simulink model "bot_demo_org"  (Simulink 10.0)
settings: Solver=ode45  StartTime=0.0  StopTime=inf  FixedStep=0.1  RelTol=1e-3
undefined symbols (not defined in the file): C_l_be, C_l_p, C_l_r, C_l_xi, C_l_ze, C_Q_be, C_Q_p, C_Q_r, C_Q_xi, C_Q_ze
settings Model: Creator=jjbuchholz  LastModifiedBy=annonymous  ExtModeTrigMode=oneshot  ExtModeArmWhenConnect=off
settings DataIOCC: ExternalInput=[0 43068.267045196386 0 -0.018368082169447898 0 199.99999999999997 0 0.05890055295549914 0 0 0]  FinalStateName=xfinal  InitialState=[0;0.05890055295549914;0;0;0;0;199.65317277347208;0;11.773300365067556;0;0;0;0;0;0;43068.267045196386;43068.267045196386;43068.267045196386;43068.267045196386]  LoadExternalInput=on  LoadInitialState=on  SignalLoggingSaveFormat=ModelDataLogs  SignalLoggingName=sigsOut
settings OptimizationCC: BlockReduction=off  BooleanDataType=off  ExpressionDepthLimit=2147483647
settings DebuggingCC: SaveWithParameterizedLinksMsg=none  SignalResolutionControl=TryResolveAllWithWarning  MultiTaskDSMMsg=warning  MultiTaskCondExecSysMsg=none  FcnCallInpInsideContextMsg=warning  StateNameClashWarn=warning  InitInArrayFormatMsg=none
settings HardwareCC: TargetUnknown=on
settings GRTTargetCC: GeneratePreprocessorConditionals=Disable all
settings ConfigComp: CovExternalEMLEnable=off

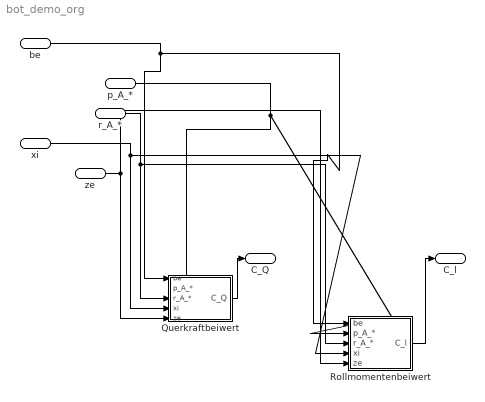
== system bot_demo_org ==
  be : Inport
  p_A_* : Inport  Port=2
  r_A_* : Inport  Port=3
  xi : Inport  Port=4
  ze : Inport  Port=5
  Querkraftbeiwert : Subsystem
  Rollmomentenbeiwert : Subsystem
  C_Q : Outport  InitialOutput=0
  C_l : Outport  Port=2  InitialOutput=0
  wires:
  Querkraftbeiwert/1(C_Q) -> C_Q/1
  Rollmomentenbeiwert/1(C_l) -> C_l/1
  ze/1 -> Querkraftbeiwert/5(ze), Rollmomentenbeiwert/5(ze)
  xi/1 -> Rollmomentenbeiwert/4(xi), Querkraftbeiwert/4(xi)
  r_A_*/1 -> Querkraftbeiwert/3(r_A_*), Rollmomentenbeiwert/3(r_A_*)
  p_A_*/1 -> Rollmomentenbeiwert/2(p_A_*), Querkraftbeiwert/2(p_A_*)
  be/1 -> Querkraftbeiwert/1(be), Rollmomentenbeiwert/1(be)

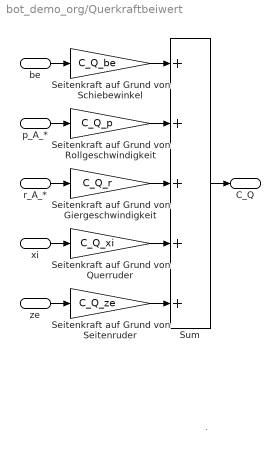
== system bot_demo_org/Querkraftbeiwert ==
  note: .
  be : Inport
  p_A_* : Inport  Port=2
  r_A_* : Inport  Port=3
  xi : Inport  Port=4
  ze : Inport  Port=5
  Seitenkraft auf Grund von Giergeschwindigkeit : Gain  Gain=C_Q_r  SaturateOnIntegerOverflow=on  OutDataTypeStr=Inherit: Same as input  ParamDataTypeStr=Inherit: Same as input
  Seitenkraft auf Grund von Querruder : Gain  Gain=C_Q_xi  SaturateOnIntegerOverflow=on  OutDataTypeStr=Inherit: Same as input  ParamDataTypeStr=Inherit: Same as input
  Seitenkraft auf Grund von Rollgeschwindigkeit : Gain  Gain=C_Q_p  SaturateOnIntegerOverflow=on  OutDataTypeStr=Inherit: Same as input  ParamDataTypeStr=Inherit: Same as input
  Seitenkraft auf Grund von Schiebewinkel : Gain  Gain=C_Q_be  SaturateOnIntegerOverflow=on  OutDataTypeStr=Inherit: Same as input  ParamDataTypeStr=Inherit: Same as input
  Seitenkraft auf Grund von Seitenruder : Gain  Gain=C_Q_ze  SaturateOnIntegerOverflow=on  OutDataTypeStr=Inherit: Same as input  ParamDataTypeStr=Inherit: Same as input
  Sum : Sum  Inputs=5  SaturateOnIntegerOverflow=on  InputSameDT=on  OutDataTypeStr=Inherit: Same as first input
  C_Q : Outport  InitialOutput=0
  wires:
  xi/1 -> Seitenkraft auf Grund von Querruder/1
  r_A_*/1 -> Seitenkraft auf Grund von Giergeschwindigkeit/1
  Sum/1 -> C_Q/1
  p_A_*/1 -> Seitenkraft auf Grund von Rollgeschwindigkeit/1
  Seitenkraft auf Grund von Querruder/1 -> Sum/4
  Seitenkraft auf Grund von Giergeschwindigkeit/1 -> Sum/3
  Seitenkraft auf Grund von Rollgeschwindigkeit/1 -> Sum/2
  Seitenkraft auf Grund von Schiebewinkel/1 -> Sum/1
  be/1 -> Seitenkraft auf Grund von Schiebewinkel/1
  ze/1 -> Seitenkraft auf Grund von Seitenruder/1
  Seitenkraft auf Grund von Seitenruder/1 -> Sum/5

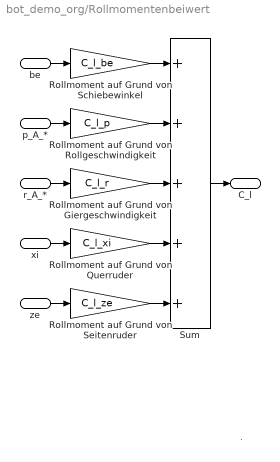
== system bot_demo_org/Rollmomentenbeiwert ==
  note: .
  be : Inport
  p_A_* : Inport  Port=2
  r_A_* : Inport  Port=3
  xi : Inport  Port=4
  ze : Inport  Port=5
  Rollmoment auf Grund von Giergeschwindigkeit : Gain  Gain=C_l_r  SaturateOnIntegerOverflow=on  OutDataTypeStr=Inherit: Same as input  ParamDataTypeStr=Inherit: Same as input
  Rollmoment auf Grund von Querruder : Gain  Gain=C_l_xi  SaturateOnIntegerOverflow=on  OutDataTypeStr=Inherit: Same as input  ParamDataTypeStr=Inherit: Same as input
  Rollmoment auf Grund von Rollgeschwindigkeit : Gain  Gain=C_l_p  SaturateOnIntegerOverflow=on  OutDataTypeStr=Inherit: Same as input  ParamDataTypeStr=Inherit: Same as input
  Rollmoment auf Grund von Schiebewinkel : Gain  Gain=C_l_be  SaturateOnIntegerOverflow=on  OutDataTypeStr=Inherit: Same as input  ParamDataTypeStr=Inherit: Same as input
  Rollmoment auf Grund von Seitenruder : Gain  Gain=C_l_ze  SaturateOnIntegerOverflow=on  OutDataTypeStr=Inherit: Same as input  ParamDataTypeStr=Inherit: Same as input
  Sum : Sum  Inputs=5  SaturateOnIntegerOverflow=on  InputSameDT=on  OutDataTypeStr=Inherit: Same as first input
  C_l : Outport  InitialOutput=0
  wires:
  Rollmoment auf Grund von Seitenruder/1 -> Sum/5
  ze/1 -> Rollmoment auf Grund von Seitenruder/1
  be/1 -> Rollmoment auf Grund von Schiebewinkel/1
  Rollmoment auf Grund von Schiebewinkel/1 -> Sum/1
  Rollmoment auf Grund von Rollgeschwindigkeit/1 -> Sum/2
  Rollmoment auf Grund von Giergeschwindigkeit/1 -> Sum/3
  Rollmoment auf Grund von Querruder/1 -> Sum/4
  p_A_*/1 -> Rollmoment auf Grund von Rollgeschwindigkeit/1
  Sum/1 -> C_l/1
  r_A_*/1 -> Rollmoment auf Grund von Giergeschwindigkeit/1
  xi/1 -> Rollmoment auf Grund von Querruder/1
